simulink model "loop"  (R2018a)
settings: Solver=ode4  StartTime=0.0  StopTime=t_end  FixedStep=t_step  RelTol=1e-3
undefined symbols (not defined in the file): C, d_delta, d_on, d_time, d_val, den, den1, E, iL0, Kp, L, n_on, num, num1, R, r_delta, r_on, r_time, r_val, sel, sigma_n, t_step, t_switch, Ti, u0, u_manual, uC0, y0
settings Model: Creator=Milosh Yokich  LastModifiedBy=Milosh Yokich

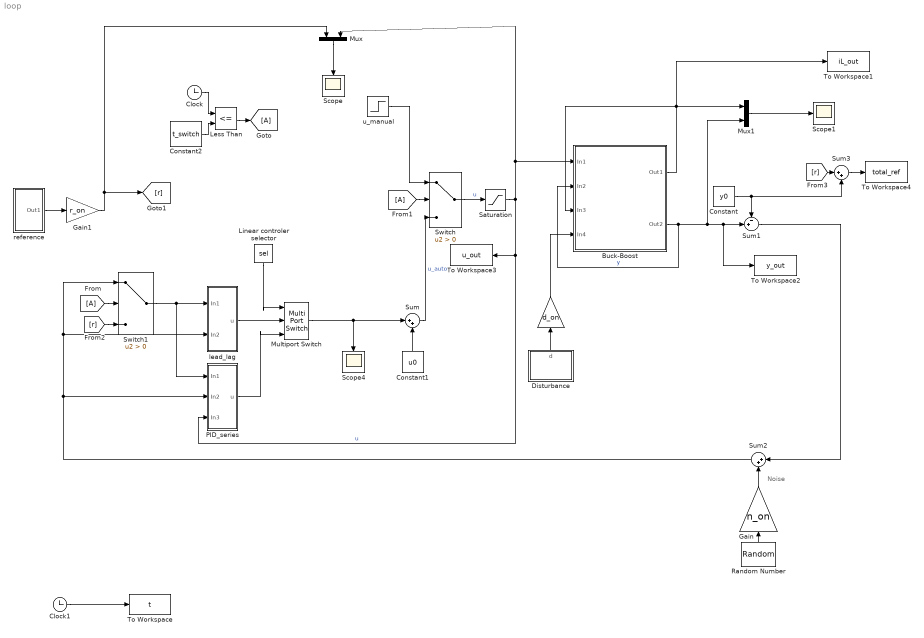
== system loop ==
  note: Noise
  " " : Gain  Gain=d_on
  Buck-Boost : Subsystem
  Clock : Clock
  Clock1 : Clock
  Constant : Constant  Value=y0
  Constant1 : Constant  Value=u0
  Constant2 : Constant  Value=t_switch
  Disturbance : Subsystem
  Gain : Gain  Gain=n_on
  Gain1 : Gain  Gain=r_on
  Less Than : RelationalOperator  Operator=<=  OutDataTypeStr=boolean  ZeroCross=off  RndMeth=Simplest
  Linear controler selector : Constant  Value=sel  VectorParams1D=off  SampleTime=-1
  Multiport Switch : MultiPortSwitch  Inputs=2
  Mux : Mux  Inputs=2
  Mux1 : Mux  Inputs=2
  "PID_series " : Subsystem
  Random Number : RandomNumber  Variance=sigma_n  SampleTime=t_step
  Saturation : Saturate  UpperLimit=1  LowerLimit=0
  Scope : Scope
  Scope1 : Scope
  Scope4 : Scope
  Sum : Sum  Inputs=|++
  Sum1 : Sum  Inputs=-+|
  Sum2 : Sum  Inputs=|++
  Sum3 : Sum  Inputs=|++
  Switch : Switch  Criteria=u2 > Threshold
  Switch1 : Switch  Criteria=u2 > Threshold
  To Workspace : ToWorkspace  VariableName=t  SampleTime=-1
  To Workspace1 : ToWorkspace  VariableName=iL_out  SampleTime=-1
  To Workspace2 : ToWorkspace  VariableName=y_out  SampleTime=-1
  To Workspace3 : ToWorkspace  VariableName=u_out  SampleTime=-1
  To Workspace4 : ToWorkspace  VariableName=total_ref  SampleTime=-1
  "lead_lag " : Subsystem
  "reference " : Subsystem
  "u_manual " : Step  Time=0  After=u_manual  SampleTime=0
  wires:
  Random Number/1 -> Gain/1
  Constant/1 -> Sum1/1, Sum3/2
  Sum/1 -> Switch/3  "u_auto"
  "u_manual "/1 -> Switch/1
  Buck-Boost/1(Out1) -> Buck-Boost/3(In3), Mux1/1, To Workspace1/1
  Clock1/1 -> To Workspace/1
  Mux/1 -> Scope/1
  Mux1/1 -> Scope1/1
  Linear controler selector/1 -> Multiport Switch/1
  Saturation/1 -> "PID_series "/3(In3), To Workspace3/1, Buck-Boost/1(In1), Mux/2  "u"
  Switch/1 -> Saturation/1  "u"
  "lead_lag "/1(u) -> Multiport Switch/2
  [A] -> Switch1/2
  Clock/1 -> Less Than/1
  Less Than/1 -> [A]
  Constant2/1 -> Less Than/2
  [A] -> Switch/2
  [r] -> Switch1/3
  [r] -> Sum3/1
  Sum3/1 -> To Workspace4/1
  Gain1/1 -> [r], Mux/1
  Disturbance/1(d) -> " "/1
  "reference "/1(Out1) -> Gain1/1
  Sum1/1 -> Sum2/1
  Gain/1 -> Sum2/2
  Buck-Boost/2(Out2) -> Buck-Boost/2(In2), Mux1/2, Sum1/2, To Workspace2/1  "y"
  Multiport Switch/1 -> Sum/1, Scope4/1
  Sum2/1 -> "PID_series "/2(In2), Switch1/1, "lead_lag "/2(In2)
  Switch1/1 -> "PID_series "/1(In1), "lead_lag "/1(In1)
  Constant1/1 -> Sum/2
  "PID_series "/1(u) -> Multiport Switch/3
  " "/1 -> Buck-Boost/4(In4)

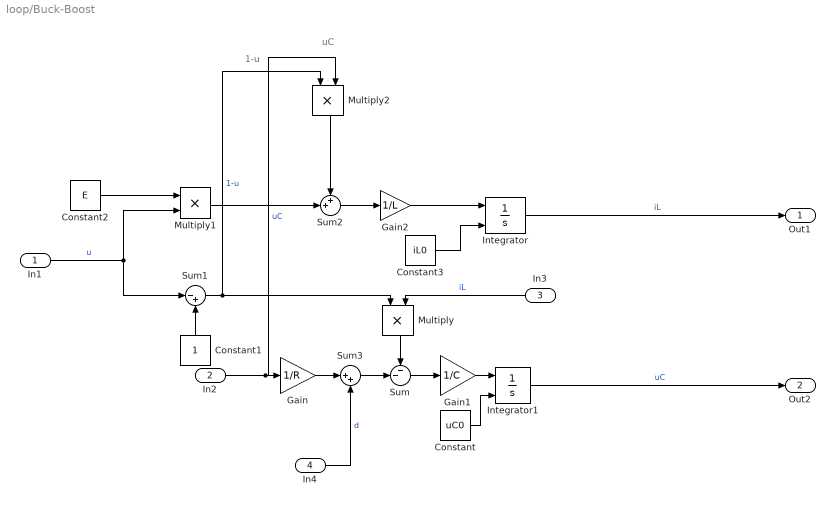
== system loop/Buck-Boost ==
  note: uC
  note: 1-u
  In1 : Inport
  In2 : Inport  Port=2
  In3 : Inport  Port=3
  In4 : Inport  Port=4
  Constant : Constant  Value=uC0
  Constant1 : Constant
  Constant2 : Constant  Value=E
  Constant3 : Constant  Value=iL0
  Gain : Gain  Gain=1/R
  Gain1 : Gain  Gain=1/C
  Gain2 : Gain  Gain=1/L
  Integrator : Integrator  InitialConditionSource=external
  Integrator1 : Integrator  InitialConditionSource=external
  Multiply : Product
  Multiply1 : Product
  Multiply2 : Product
  Sum : Sum  Inputs=--|
  Sum1 : Sum  Inputs=|-+
  Sum2 : Sum  Inputs=++|
  Sum3 : Sum  Inputs=|++
  Out1 : Outport
  Out2 : Outport  Port=2
  wires:
  In4/1 -> Sum3/2  "d"
  Sum3/1 -> Sum/2
  Gain/1 -> Sum3/1
  In3/1 -> Multiply/2  "iL"
  In2/1 -> Gain/1, Multiply2/2  "uC"
  Sum2/1 -> Gain2/1
  Sum/1 -> Gain1/1
  Constant/1 -> Integrator1/2
  Constant1/1 -> Sum1/2
  Multiply/1 -> Sum/1
  Constant3/1 -> Integrator/2
  In1/1 -> Sum1/1, Multiply1/2  "u"
  Multiply1/1 -> Sum2/2
  Gain1/1 -> Integrator1/1
  Integrator/1 -> Out1/1  "iL"
  Gain2/1 -> Integrator/1
  Sum1/1 -> Multiply2/1, Multiply/1  "1-u"
  Integrator1/1 -> Out2/1  "uC"
  Constant2/1 -> Multiply1/1
  Multiply2/1 -> Sum2/1

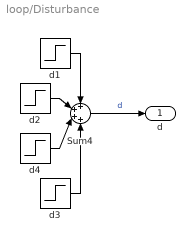
== system loop/Disturbance ==
  Sum4 : Sum  Inputs=++++
  "d1 " : Step  Time=d_time  After=d_val  SampleTime=0
  "d2 " : Step  Time=d_time + d_delta  After=-d_val  SampleTime=0
  "d3 " : Step  Time=d_time + d_delta*2  After=-d_val  SampleTime=0
  "d4 " : Step  Time=d_time + d_delta*3  After=d_val  SampleTime=0
  d : Outport
  wires:
  "d3 "/1 -> Sum4/4
  "d1 "/1 -> Sum4/1
  "d2 "/1 -> Sum4/2
  "d4 "/1 -> Sum4/3
  Sum4/1 -> d/1  "d"

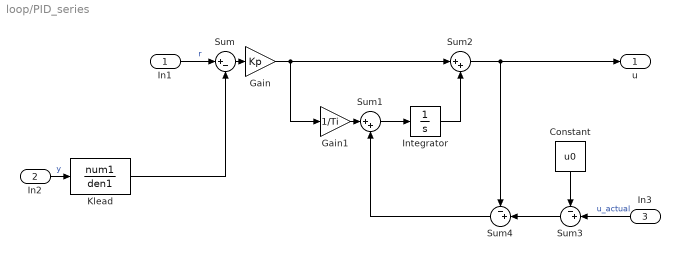
== system loop/PID_series  ==
  In1 : Inport
  In2 : Inport  Port=2
  In3 : Inport  Port=3
  Constant : Constant  Value=u0
  Gain : Gain  Gain=Kp
  Gain1 : Gain  Gain=1/Ti
  Integrator : Integrator
  Klead : TransferFcn  Numerator=num1  Denominator=den1
  Sum : Sum  Inputs=|+-
  Sum1 : Sum  Inputs=|++
  Sum2 : Sum  Inputs=|++
  Sum3 : Sum  Inputs=-+|
  Sum4 : Sum  Inputs=-+|
  u : Outport
  wires:
  In1/1 -> Sum/1  "r"
  In2/1 -> Klead/1  "y"
  Klead/1 -> Sum/2
  Sum/1 -> Gain/1
  Sum1/1 -> Integrator/1
  Gain1/1 -> Sum1/1
  Gain/1 -> Sum2/1, Gain1/1
  Integrator/1 -> Sum2/2
  Sum2/1 -> Sum4/1, u/1
  In3/1 -> Sum3/2  "u_actual"
  Sum3/1 -> Sum4/2
  Constant/1 -> Sum3/1
  Sum4/1 -> Sum1/2

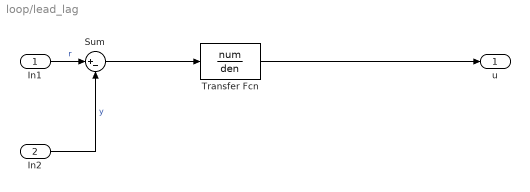
== system loop/lead_lag  ==
  In1 : Inport
  In2 : Inport  Port=2
  Sum : Sum  Inputs=|+-
  Transfer Fcn : TransferFcn  Numerator=num  Denominator=den
  u : Outport
  wires:
  In2/1 -> Sum/2  "y"
  In1/1 -> Sum/1  "r"
  Sum/1 -> Transfer Fcn/1
  Transfer Fcn/1 -> u/1

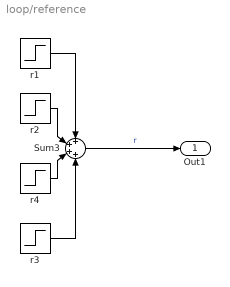
== system loop/reference  ==
  Sum3 : Sum  Inputs=++++
  "r1 " : Step  Time=r_time  After=r_val  SampleTime=0
  "r2 " : Step  Time=r_time + r_delta  After=-r_val  SampleTime=0
  "r3 " : Step  Time=r_time + 2*r_delta  After=-r_val  SampleTime=0
  "r4 " : Step  Time=r_time + 3*r_delta  After=r_val  SampleTime=0
  Out1 : Outport
  wires:
  Sum3/1 -> Out1/1  "r"
  "r2 "/1 -> Sum3/2
  "r3 "/1 -> Sum3/4
  "r4 "/1 -> Sum3/3
  "r1 "/1 -> Sum3/1
